simulink model "rip"  (R2025b)
settings: Solver=ode4  StartTime=0.0  StopTime=1.5  FixedStep=0.001  MaxStep=0.001  RelTol=1e-3
model workspace (MAT data in the model file):
  ba = Simulink.Parameter
  ba.Value = 0.005
  ba.Complexity = 'real'
  ba.Dimensions = [1 1]
  ba.DataType = 'auto'
  bp = Simulink.Parameter
  bp.Value = 0.0007
  bp.Complexity = 'real'
  bp.Dimensions = [1 1]
  bp.DataType = 'auto'
  g = Simulink.Parameter
  g.Value = 9.81
  g.Complexity = 'real'
  g.Dimensions = [1 1]
  g.DataType = 'auto'
  la = Simulink.Parameter
  la.Value = 0.155
  la.Complexity = 'real'
  la.Dimensions = [1 1]
  la.DataType = 'auto'
  lp = Simulink.Parameter
  lp.Value = 0.155
  lp.Complexity = 'real'
  lp.Dimensions = [1 1]
  lp.DataType = 'auto'
  ma = Simulink.Parameter
  ma.Value = 0.21
  ma.Complexity = 'real'
  ma.Dimensions = [1 1]
  ma.DataType = 'auto'
  mp = Simulink.Parameter
  mp.Value = 0.156
  mp.Complexity = 'real'
  mp.Dimensions = [1 1]
  mp.DataType = 'auto'
libraries: eeGeneralControl x2
settings Model: Creator=hasza  LastModifiedBy=detective
settings SolverCC: NumberNewtonIterations=200.0  ZeroCrossControl=EnableAll  MaxZcPerStep=100.0  MaxZcBracketingIterations=100.0
settings OptimizationCC: DefaultParameterBehavior=Inlined  UseDivisionForNetSlopeComputation=on  GainParamInheritBuiltInType=on  UseFloatMulNetSlope=on  InlineInvariantSignals=on  PassReuseOutputArgsAs=Individual arguments  ZeroExternalMemoryAtStartup=off  ZeroInternalMemoryAtStartup=off  NoFixptDivByZeroProtection=on  EfficientFloat2IntCast=on  LifeSpan=1  OptimizeBlockOrder=speed  DifferentSizesBufferReuse=on  EfficientTunableParamExpr=on
settings DebuggingCC: ParameterTunabilityLossMsg=error
settings HardwareCC: ProdBitPerPointer=32.0  ProdBitPerSizeT=32.0  ProdBitPerPtrDiffT=32.0  ProdLargestAtomicInteger=Long  ProdWordSize=32.0  ProdLongLongMode=on  ProdHWDeviceType=ARM Compatible->ARM 10
settings SFSimCC: MATLABDynamicMemAlloc=off
settings RTWCC: SystemTargetFile=ert.tlc  GenCodeOnly=on  TemplateMakefile=ert_default_tmf  Description=Embedded Coder
settings CodeAppCC: ForceParamTrailComments=on  IgnoreCustomStorageClasses=off  OperatorAnnotations=on  SimulinkDataObjDesc=on  SFDataObjDesc=on  CustomSymbolStrGlobalVar=rt$N$M  CustomSymbolStrType=$N$M  CustomSymbolStrFcn=$N$M$F  CustomSymbolStrMacro=$N$M  InsertBlockDesc=on
settings ERTTargetCC: ERTCustomFileTemplate=example_file_process.tlc  ERTFilePackagingFormat=CompactWithDataFile  TargetLangStandard=C99 (ISO)  GenerateSampleERTMain=on  IncludeMdlTerminateFcn=off  CombineSignalStateStructs=on  SupportAbsoluteTime=off  SupportComplex=off  SupportContinuousTime=on  SupportNonInlinedSFcns=on
settings SimscapeCC: SimscapeLogDecimation=1  SimscapeLogDataHistory=5000

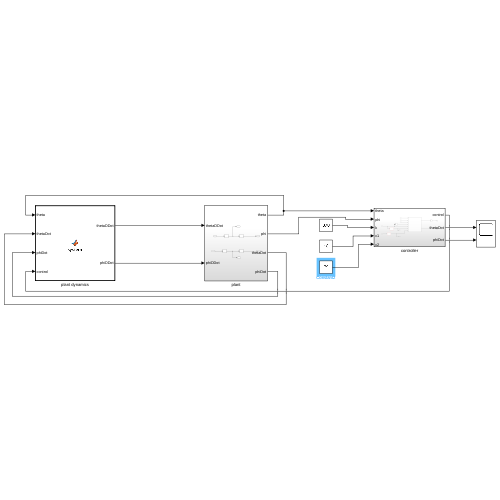
[thumbnail: Simulink's stored preview of the top-level diagram]
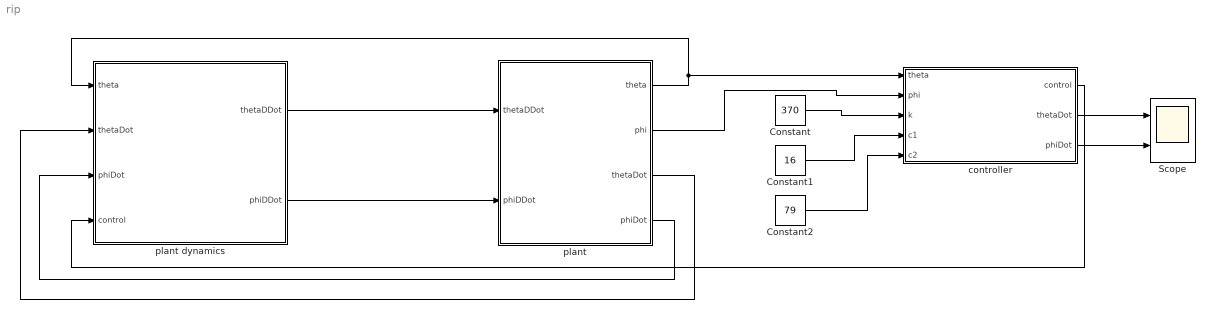
== system rip ==
  Constant : Constant  Value=370
  Constant1 : Constant  Value=16
  Constant2 : Constant  Value=79
  Scope : Scope  NumInputPorts=2
      settings: ActiveDisplayYMinimum=-7.15817  ActiveDisplayYMaximum=9.05136
  controller : Subsystem
  plant : Subsystem
  plant dynamics : MATLAB Function  TreatAsAtomicUnit=on
  wires:
  plant/1(theta) -> plant dynamics/1(theta), controller/1(theta)
  plant/2(phi) -> controller/2(phi)
  controller/1(control) -> plant dynamics/4(control)
  plant/4(phiDot) -> plant dynamics/3(phiDot)
  plant/3(thetaDot) -> plant dynamics/2(thetaDot)
  plant dynamics/1(thetaDDot) -> plant/1(thetaDDot)
  plant dynamics/2(phiDDot) -> plant/2(phiDDot)
  controller/2(thetaDot) -> Scope/1
  controller/3(phiDot) -> Scope/2
  Constant/1 -> controller/3(k)
  Constant1/1 -> controller/4(c1)
  Constant2/1 -> controller/5(c2)

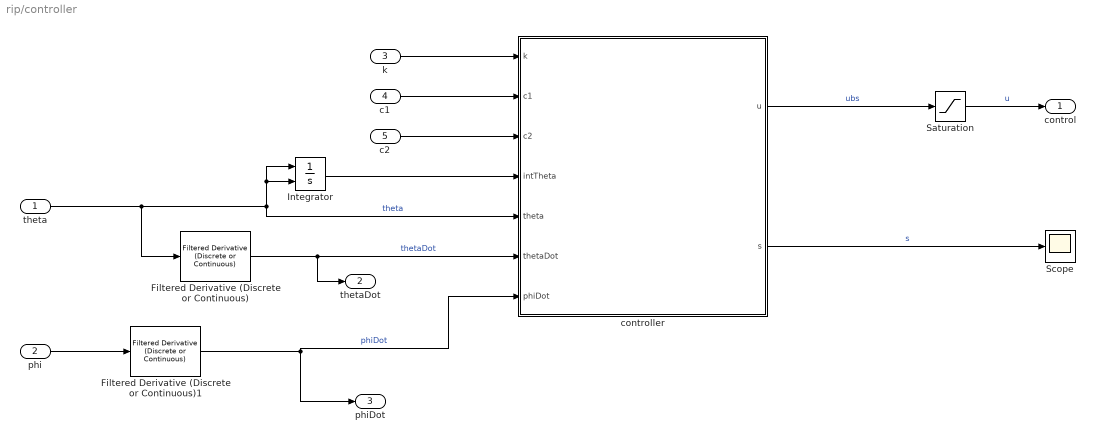
== system rip/controller ==
  theta : Inport
  phi : Inport  Port=2
  k : Inport  Port=3
  c1 : Inport  Port=4
  c2 : Inport  Port=5
  Filtered Derivative (Discrete or Continuous) : eeGeneralControl/Filtered Derivative (Discrete or Continuous)  K=1  T=0.0001  B=inf  A=-inf  minRatio=10  init_option=Inherited from block input  x0=0  Ts=-1
      settings: LibrarySourceBlock=|
      | ee_sl_lib/General Control/Filtered Derivative
      | (Discrete or Continuous)
  Filtered Derivative (Discrete or Continuous)1 : eeGeneralControl/Filtered Derivative (Discrete or Continuous)  K=1  T=0.0001  B=inf  A=-inf  minRatio=10  init_option=Inherited from block input  x0=0  Ts=-1
      settings: LibrarySourceBlock=|
      | ee_sl_lib/General Control/Filtered Derivative
      | (Discrete or Continuous)
  Integrator : Integrator  ExternalReset=either  WrapState=on  WrappedStateUpperValue=3.14  WrappedStateLowerValue=-3.14
  Saturation : Saturate  UpperLimit=2  LowerLimit=-2
  Scope : Scope
  controller : MATLAB Function  TreatAsAtomicUnit=on
  control : Outport
  thetaDot : Outport  Port=2
  phiDot : Outport  Port=3
  wires:
  theta/1 -> Filtered Derivative (Discrete or Continuous)/1, Integrator/2, Integrator/1, controller/5(theta)  "theta"
  phi/1 -> Filtered Derivative (Discrete or Continuous)1/1
  Saturation/1 -> control/1  "u"
  Filtered Derivative (Discrete or Continuous)/1 -> thetaDot/1, controller/6(thetaDot)  "thetaDot"
  Filtered Derivative (Discrete or Continuous)1/1 -> phiDot/1, controller/7(phiDot)  "phiDot"
  controller/1(u) -> Saturation/1  "ubs"
  Integrator/1 -> controller/4(intTheta)
  controller/2(s) -> Scope/1  "s"
  k/1 -> controller/1(k)
  c1/1 -> controller/2(c1)
  c2/1 -> controller/3(c2)

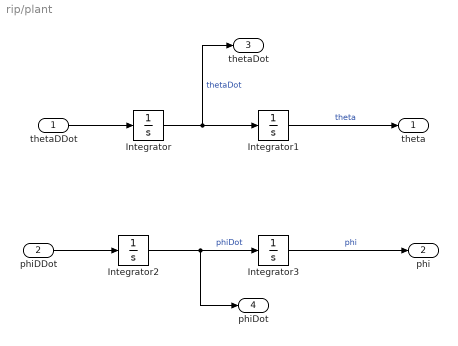
== system rip/plant ==
  thetaDDot : Inport
  phiDDot : Inport  Port=2
  Integrator : Integrator
  Integrator1 : Integrator  InitialCondition=0.6
  Integrator2 : Integrator
  Integrator3 : Integrator
  theta : Outport
  phi : Outport  Port=2
  thetaDot : Outport  Port=3
  phiDot : Outport  Port=4
  wires:
  Integrator/1 -> thetaDot/1, Integrator1/1  "thetaDot"
  Integrator2/1 -> Integrator3/1, phiDot/1  "phiDot"
  Integrator1/1 -> theta/1  "theta"
  Integrator3/1 -> phi/1  "phi"
  thetaDDot/1 -> Integrator/1
  phiDDot/1 -> Integrator2/1

== matlab function rip/plant dynamics ==
  data: theta input; thetaDDot output; thetaDot input; phiDot input; phiDDot output; control input
function [thetaDDot, phiDDot] = system(theta, thetaDot, phiDot, control)
% SMC Controller for Rotating Inverted Pendulum

% System Parameters (needed for control calculation)
% Physical parameters
ma = 0.21;      % Arm mass (kg)
mp = 0.156;    % Pendulum mass (kg)
la = 0.155;    % Arm length (m)
lp = 0.155;    % Pendulum length (m)
ba = 0.005;    % Arm damping coefficient (N·m·s/rad)
bp = 0.0007;   % Pendulum damping coefficient (N·m·s/rad)
g = 9.81;      % Gravity (m/s²)

% Derived parameters
p1 = (1/3 * ma + mp) * la^2;
p2 = (1/4 * mp) * lp^2;
p3 = (1/2 * mp) * lp * la;
p4 = (1/2 * mp) * lp * g;
p5 = (1/12 * mp) * lp^2;


% Mass Matrix Elements
m11 = p1 + p2 * sin(theta)^2;
m12 = p3 * cos(theta);
m22 = p2 + p5;

% Nonlinear terms (Coriolis, centrifugal, gravity, friction)
H1 = p2 * sin(2*theta) * thetaDot * phiDot ...
     - p3 * sin(theta) * thetaDot^2 ...      
     + ba * phiDot;                           

H2 = -0.5 * p2 * sin(2*theta) * phiDot^2 ...  
      - p4 * sin(theta) ...                  
      + bp * thetaDot;

% Avoid division by zero
threshold = 1e-5;
if abs(m12) < threshold
     m12 = threshold * sign(m12);  % Preserves sign
end

% Calculate Control Input
detM = m11 * m22 - m12^2;

phiDDot = (m22*(control - H1) + m12*H2)/detM;

thetaDDot = (m12*(H1 - control) - m11*H2)/detM;

end

== matlab function rip/controller/controller ==
  data: k input; c1 input; c2 input; intTheta input; theta input; u output; thetaDot input; phiDot input; s output
function [u, s] = smcController(k, c1, c2, intTheta, theta, thetaDot, phiDot)
% SMC Controller for Rotating Inverted Pendulum
% Inputs: theta (pendulum angle), thetaDot (pendulum velocity), phiDot (arm velocity)
% Output: tauPhi (control torque)


% Physical parameters
ma = 0.21; % Arm mass (kg)
mp = 0.156; % Pendulum mass (kg)
la = 0.155; % Arm length (m)
lp = 0.155; % Pendulum length (m)
ba = 0.005; % Arm damping coefficient (N·m·s/rad)
bp = 0.0007; % Pendulum damping coefficient (N·m·s/rad)
g = 9.81; % Gravity (m/s²)


% Derived parameters
p1 = (1/3 * ma + mp) * la^2;
p2 = (1/4 * mp) * lp^2;
p3 = (1/2 * mp) * lp * la;
p4 = (1/2 * mp) * lp * g;
p5 = (1/12 * mp) * lp^2;

% Calculate Sliding Surface
s = thetaDot + c1 * theta + c2* intTheta;

% Adaptive boundary layer based on angle and sliding surface
n = 0.1 + 0.5*abs(theta) + 0.1*abs(s);
n = min(n, 0.8); % Cap the boundary layer

% Mass Matrix Elements
m11 = p1 + p2 * sin(theta)^2;
m12 = p3 * cos(theta);
m22 = p2 + p5;

% Nonlinear terms (Coriolis, centrifugal, gravity, friction)
H1 = p2 * sin(2*theta) * thetaDot * phiDot ...
 - p3 * sin(theta) * thetaDot^2 ...
 + ba * phiDot;
H2 = -0.5 * p2 * sin(2*theta) * phiDot^2 ...
 - p4 * sin(theta) ...
 + bp * thetaDot;

% Avoid division by zero
threshold = 1e-5;
if abs(m12) < threshold
 m12 = threshold * sign(m12); % Preserves sign
end

% Calculate Control Input
detM = m11 * m22 - m12^2;
% Control gain (effect of tauPhi on thetaDDot)
gControl = m12 / detM;
% Drift dynamics (effect of nonlinear terms on thetaDDot)
f = (m12*H1 - m11*H2) / detM;

% Equivalent control
uEq = (f + c1 * thetaDot + c2* theta) / gControl;
% Complete control law: equivalent control + switching control
uSMC = uEq + (k / gControl) * sqrt(abs(s)) * tanh(s / n);

% Bang-bang swing-up control
% Simple position-based bang-bang to move pendulum left/right
if theta > 0
    uBB = -2.0; % Push left when pendulum is on right side
else
    uBB = 2.0;  % Push right when pendulum is on left side
end

% Control mode switching
if abs(theta) >= 0.8
    u = uBB;
else
    u = uSMC;
end
end
